simulink model "Test_ISA"  (R2024b)
settings: Solver=VariableStepAuto  StartTime=0.0  StopTime=10.0  RelTol=1e-3
libraries: Atmospheric x2
settings Model: Creator=ada09  LastModifiedBy=ada09

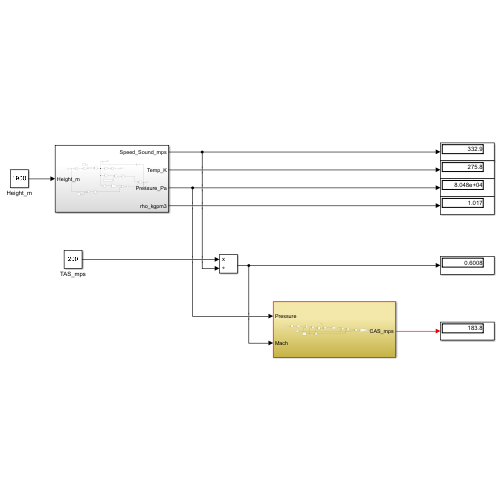
[thumbnail: Simulink's stored preview of the top-level diagram]
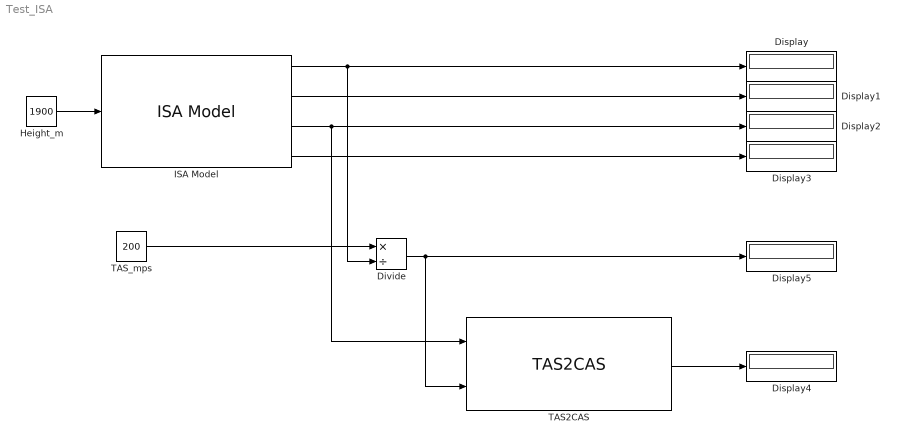
== system Test_ISA ==
  Display{,1..5} (6 alike) : Display
  Divide : Product  Inputs=*/
  Height_m : Constant  Value=1900
  ISA Model : Atmospheric/ISA Model  SystemSampleTime=-1  VariantActivationTime=update diagram  AllowFlexibleInterface=on  Latency=0  AutoFrameSizeCalculation=off
  TAS2CAS : Atmospheric/TAS2CAS  SystemSampleTime=-1  VariantActivationTime=update diagram  AllowFlexibleInterface=on  Latency=0  AutoFrameSizeCalculation=off
  TAS_mps : Constant  Value=200
  wires:
  ISA Model/3 -> Display2/1, TAS2CAS/1
  ISA Model/4 -> Display3/1
  Divide/1 -> Display5/1, TAS2CAS/2
  TAS2CAS/1 -> Display4/1
  TAS_mps/1 -> Divide/1
  ISA Model/2 -> Display1/1
  Height_m/1 -> ISA Model/1
  ISA Model/1 -> Display/1, Divide/2
